simulink model "es3_ACPC_sim"  (R2022b)
settings: Solver=VariableStepAuto  StartTime=0.0  StopTime=10.0  RelTol=1e-3
values from neighbouring files (symbols this model uses):
  r = -1:0.2:1    [ES3.m]
undefined symbols (not defined in the file or in its folder): j
settings Model: Creator=claudio  LastModifiedBy=claudio
settings SolverCC: AlgebraicLoopSolver=TrustRegion
settings DebuggingCC: UnconnectedInputMsg=warning  UnconnectedOutputMsg=warning  UnconnectedLineMsg=warning  SFMachineParentedDataDiag=warning
settings ModelReferenceCC: EnableRefExpFcnMdlSchedulingChecks=on
settings RTWCC: DLArmComputeVersion=19.05

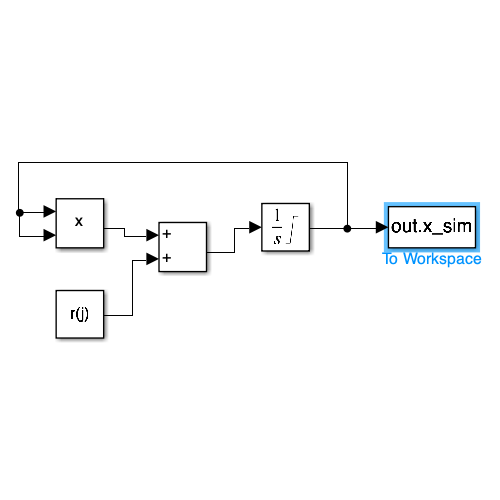
[thumbnail: Simulink's stored preview of the top-level diagram]
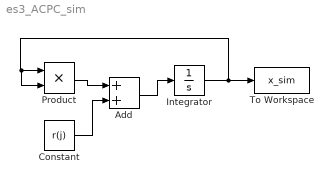
== system es3_ACPC_sim ==
  Add : Sum
  Constant : Constant  Value=r(j)
  Integrator : Integrator  InitialCondition=-4  LimitOutput=on  UpperSaturationLimit=10  LowerSaturationLimit=-10
  Product : Product
  To Workspace : ToWorkspace  VariableName=x_sim  SampleTime=-1
  wires:
  Product/1 -> Add/1
  Add/1 -> Integrator/1
  Integrator/1 -> To Workspace/1, Product/2, Product/1
  Constant/1 -> Add/2
